simulink model "TempCtrl"  (R2026a)
settings: Solver=ode3  StopTime=Inf  FixedStep=0.005
PostLoadFcn:
  | addpath(fullfile(fileparts(get_param(bdroot,'FileName')),'helpers')); TempCtrlParameters;
values from neighbouring files (symbols this model uses):
  Kp = 50    [TempCtrlParameters.m]
  SetpointDefault = 37    [TempCtrlParameters.m]
  Tn = 200    [TempCtrlParameters.m]
libraries: simulink x1
settings Model: MinMaxOverflowLogging=ForceOff  TCT_EXTMODE_CONNECTEDMODULEALLOWSEC=ON  ModifiedByFormat=Beckhoff Automation GmbH & Co. KG  SimulationMode=external  ParamWorkspaceSource=ReferencedWorkspace  Creator=Beckhoff Automation GmbH & Co. KG  LastModifiedBy=Beckhoff Automation GmbH & Co. KG
settings DataIOCC: SaveFormat=Structure  SignalLoggingSaveFormat=ModelDataLogs
settings OptimizationCC: OptimizeBlockIOStorage=off  BufferReuse=off  LocalBlockOutputs=off
settings DebuggingCC: UnderspecifiedInitializationDetection=Classic
settings HardwareCC: ProdHWDeviceType=32-bit Generic
settings SFSimCC: UsePrecompiledLibraries=Avoid  SimTargetLang=C++
settings RTWCC: SystemTargetFile=TwinCatGrt.tlc  GenCodeOnly=on  GenerateMakefile=off  TemplateMakefile=tcgrt_msbuild.tmf  GenerateReport=on  RTWVerbose=off  RetainRTWFile=on  TargetLang=C++  Description=TwinCAT GRT Target
settings CodeAppCC: MaxIdLength=50.0
settings STFCustomTargetCC: SystemTargetFile=TwinCatGrt.tlc  MultiwordLength=2048.0  ConcurrentExecutionCompliant=on  CombineOutputUpdateFcns=on  CodeInterfacePackaging=Reusable function  CPPClassGenCompliant=on  GRTInterface=off  GenerateAllocFcn=on  TcProject_Generate=on  TcProject_LowestCompatibleTcBuild=$<TwinCAT:Version:BUILD>  TcProject_LibraryCategories=$<VendorName>  TcProject_InstallPlcLibrary=off  TcProject_ProductName=$<ModuleGenerator:ProductId> $<ModuleGenerator:Version:MAJOR.MINOR>  TcProject_Versioning=Versioned  TcProject_ClassFactoryName=$<Project:Name>  TcProject_VersionSrc=$<LatestTMFile>  TcProject_Copyright=Copyright $<VendorName> $<LocalDateTime:%Y>  TcCom_Generate=on  TcProject_Description=TwinCAT executable file, generated by TwinCAT $<ModuleGenerator:ProductId>  TcProject_VendorName=TE140x Module Vendor  TcProject_VendorIcon=$<TE140x:Icon>  TcProject_IncrementVersion=Revision  TcCom_InitExceptionHandling=CallerExceptions  TcProject_DrvFileVersion=$<VersionFromFile>  TcProject_DrvProductVersion=$<DrvFileVersion>  TcProject_UseDataExchangeModules=off  TcProject_MaxVisibleArrayElements=200U  TcProject_CreateUniqueEnumItemNames=off  TcProject_CreateScopedEnums=Auto  TcCom_TcComWrapperFb=off  TcProject_CoderCppNamespace=coder  TcProject_UseIntrinsics=on  TcProject_DataExchangeModulesVersion=$<ModuleGenerator:DataExchange:Version>  TcProject_UseCodeInfoExporter=on  TcCom_ExecutionSequence=UpdateBeforeOutputMapping  TcProject_PreferIntOverLong=off  TcProject_UseStaticStlString=off  TcCom_CallerVerification=Default  TcProject_StaticStlStringCapacity=Auto  TcProject_UseCodeDescriptor=on  TcProject_PreferToolArchitectureX64=on  TcProject_UseNativeBlockDiagramExport=off  TcCom_BlockDiagramExport=on  TcProject_UseDescriptorCodeType=on  TcProject_UseLLVMCodeInfo=on  TcProject_IgnorePseudoArrayDimensions=off  TcCom_ExecutionInfoParam=on  TcProject_BuildSystem=Auto  TcProject_EnableNewPlatforms=off  TcProject_Publish=on  TcProject_CppLanguageStandard=Default  TcProject_CLanguageStandard=Default  TcProject_Verbosity=Normal  TcProject_PublishPlatformtoolset=Auto  TcProject_PublishTcOSx64E=off  TcProject_PublishConfiguration=Release  TcProject_PublishTcRTx86=on  TcProject_PublishTcRTx64=on  TcProject_PublishTcOSx64=on  TcProject_PublishTcUMx64=off  TcProject_PublishTcOSARMv8A=off  TcProject_ForceRebuildForPublish=off  TcProject_PublishTcOSARMv7A=off  TcProject_PublishTcOSARMv7M=off  TcProject_PublishTcUMx86=off  TcProject_SignTwinCatCertName=Beckhoff_N.A. (new 4024 with CPP singing).tccert  TcCom_ParametersCreateSymbols=on  TcProject_PublishParallel=on  TcProject_BuildWithWdk=inherit default  TcCom_ParametersInitValues=on  TcProject_UseTmxExtension=Auto  TcProject_SignWithTwinCatCertificate=inherit default  TcCom_BlockIoCreateSymbols=on  TcProject_TmxInstall=on  TcProject_TmxArchive=$<Project:Dir>\..\..\twincat\modules\$<Project:Name>.exe  TcCom_ContStateCreateSymbols=on  TcProject_GenerateVsSolution=No  TcProject_DeployRestart=off  TcProject_PostPublishCallbackFcn=UpdateTwinCatProjects  TcCom_DataStoreCreateSymbols=on  TcProject_LibCatPath=$<Project:Dir>\$<Project:Name>.libcat.xml  TcProject_PlcVarPrefixes=PVOID=p | BOOL=b | BOOL32=b | DATE=d | TIME_OF_DATE=td | TIME=t | LTIME=t  TcCom_MaxInternalDataAreaParts=5U  TcProject_GeneratePlcLibrary=off  TcCom_VariableSymbolMappingCustom=$<ModelName>_U=Input|$<ModelName>_Y=Output|$<ModelName>_P=ModelParameters|$<ModelName>_B=BlockIO|$<ModelName>_DW=DWork|$<ModelName>_X=ContStates  TcProject_GenerateStructDutsWithDefaultValues=Auto  TcCom_ExtModeRtAllowExecutionCommands=off  TcCom_OnlineChange=off  TcCom_OnlineChangeRestoreDataAreas=off  TcCom_Legacy_ModuleBuildInfoParam=on  TcCom_GroupName=TE140x|Simulink Modules  TcCom_GroupDisplayName=$<GroupName>  TcCom_GroupIcon=$<TE140x:Icon>  TcCom_ModuleIcon=$<TE140x:Icon>  TcCom_UpdateExceptionHandling=CallerExceptions  TcCom_OemLicenses=$<Project:OemLicenses>  TcCom_TcComWrapperFbProperties=off  TcCom_TcComWrapperFbPropertyMonitoring=NoMonitoring  TcCom_ModuleCaller=CyclicTask  TcCom_StepSizeAdaptation=RequireMatchingTaskCycleTime  TcCom_ExecuteModelCode=on  TcCom_ResolveMaskedSubsystems=on  TcCom_ExtendSignalResolution=on  TcCom_BlockDiagramVariableAccess=AssignToParent  TcCom_BlockDiagramDebugInfoExport=on  TcCom_ExecutionInfoOutput=off  TcCom_MonitorExecutionTime=off  TcCom_AccessLockState=Auto  TcCom_InputDataAccess=Input Destination DataArea  TcCom_InputCreateSymbols=on  TcCom_InputReadOnly=off  TcCom_InputInitValues=on  TcCom_OutputDataAccess=Output Source DataArea  TcCom_OutputCreateSymbols=on  TcCom_OutputReadOnly=on  TcCom_ParametersDataAccess=Internal DataArea  TcCom_ParametersReadOnly=off  TcCom_GlobalParamDefaultSharing=Define  TcCom_BlockIoDataAccess=Internal DataArea  TcCom_BlockIoReadOnly=on  TcCom_ContStateDataAccess=Internal DataArea  TcCom_ContStateReadOnly=on  TcCom_DWorkDataAccess=Internal DataArea  TcCom_DWorkCreateSymbols=on  TcCom_DWorkReadOnly=on  TcCom_DataStoreDataAccess=None  TcCom_DataStoreReadOnly=off  TcCom_AllowDataAreaForSharedData=off  TcCom_VariableSymbolMapping=Identical  TcCom_OriginalIoBlockNames=off  TcCom_StrictAccessLock=on  TcCom_ExtModeRtWaitForStart=off  TcCom_ExtModeRtAllowForParameterChange=off  TcPlcFb_Generate=on  TcPlcFb_InitExceptionHandling=CallerExceptions  TcPlcFb_UpdateExceptionHandling=CallerExceptions  TcPlcFb_OemLicenses=$<Project:OemLicenses>  TcPlcFb_MonitorExecutionTime=off  TcPlcFb_ExtModeRtAllowExecutionCommands=off  TcPlcFb_ExtModeRtWaitForStart=off  TcPlcFb_ExtModeRtAllowForParameterChange=off
settings GRTTargetCC: ExtModeMexFile=TcExtModeClient  ParMdlRefBuildCompliant=off  CompOptLevelCompliant=off  MatFileLogging=off  CodeInterfacePackaging=Reusable function  GenerateAllocFcn=on

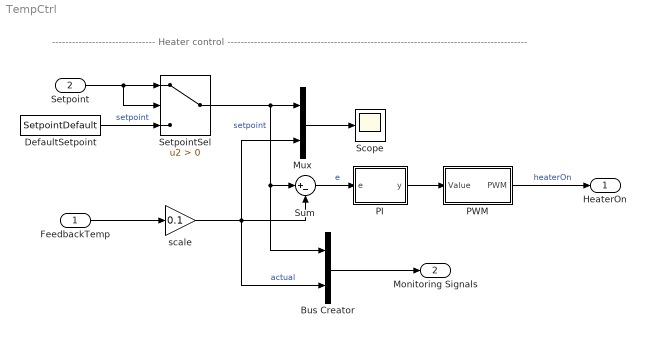
== system TempCtrl ==
  note: ------------------------------- Heater control ------------------------------------------------------------------------------------------
  FeedbackTemp : Inport  OutDataTypeStr=int16
  Setpoint : Inport  Port=2
  Bus Creator : BusCreator  Inputs=2  OutDataTypeStr=Bus: MonitoringSignalsType  NonVirtualBus=on
  DefaultSetpoint : Constant  Value=SetpointDefault
  Mux : Mux  Inputs=2
  PI : Subsystem  mask{Kp=Kp, Tn=Tn, y_min=0, y_max=60}
  PWM : Subsystem
  Scope : Scope
      settings: ActiveDisplayYMinimum=0  ActiveDisplayYMaximum=40
  SetpointSel : Switch  Criteria=u2 > Threshold  SaturateOnIntegerOverflow=off  InputSameDT=off
  Sum : Sum  Inputs=|+-
  scale : Gain  Gain=0.1  ParamDataTypeStr=double
  HeaterOn : Outport  OutDataTypeStr=boolean  VectorParamsAs1DForOutWhenUnconnected=off
  Monitoring Signals : Outport  Port=2  OutDataTypeStr=Bus: MonitoringSignalsType  VectorParamsAs1DForOutWhenUnconnected=off
  wires:
  PI/1(y) -> PWM/1(Value)
  Setpoint/1 -> SetpointSel/2, SetpointSel/1
  DefaultSetpoint/1 -> SetpointSel/3  "setpoint"
  FeedbackTemp/1 -> scale/1
  Bus Creator/1 -> Monitoring Signals/1
  scale/1 -> Sum/2, Mux/2, Bus Creator/2  "actual"
  SetpointSel/1 -> Sum/1, Bus Creator/1, Mux/1  "setpoint"
  Mux/1 -> Scope/1
  Sum/1 -> PI/1(e)  "e"
  PWM/1(PWM) -> HeaterOn/1  "heaterOn"

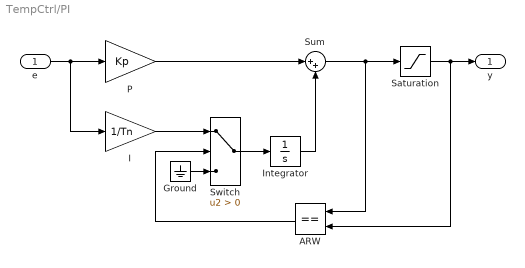
== system TempCtrl/PI ==
  e : Inport
  ARW : RelationalOperator  Operator===  OutDataTypeStr=boolean  InputSameDT=off
  Ground : Ground
  I : Gain  Gain=1/Tn
  Integrator : Integrator
  P : Gain  Gain=Kp
  Saturation : Saturate  UpperLimit=y_max  LowerLimit=y_min
  Sum : Sum  Inputs=|++
  Switch : Switch  Criteria=u2 > Threshold  SaturateOnIntegerOverflow=off  InputSameDT=off
  y : Outport  VectorParamsAs1DForOutWhenUnconnected=off
  wires:
  e/1 -> P/1, I/1
  Integrator/1 -> Sum/2
  P/1 -> Sum/1
  Sum/1 -> Saturation/1, ARW/1
  Saturation/1 -> y/1, ARW/2
  Switch/1 -> Integrator/1
  ARW/1 -> Switch/2
  I/1 -> Switch/1
  Ground/1 -> Switch/3

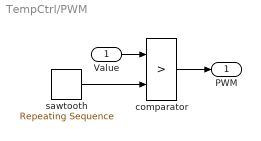
== system TempCtrl/PWM ==
  Value : Inport  OutDataTypeStr=double
  comparator : RelationalOperator  Operator=>  OutDataTypeStr=boolean  InputSameDT=off
  sawtooth : simulink/Sources/Repeating Sequence  rep_seq_t=[0 .1]  rep_seq_y=[0 60]
  PWM : Outport  OutDataTypeStr=boolean  VectorParamsAs1DForOutWhenUnconnected=off
  wires:
  Value/1 -> comparator/1
  sawtooth/1 -> comparator/2
  comparator/1 -> PWM/1
